simulink model "pole_placement_test"  (R2015b)
settings: Solver=ode3  StartTime=0.0  StopTime=10  FixedStep=0.002  RelTol=1e-3
values from neighbouring files (symbols this model uses):
  k0 = double(poly_coeffs(1))    [pole_placement_script.m]
  k1 = double(poly_coeffs(2))    [pole_placement_script.m]
  k2 = double(poly_coeffs(3))    [pole_placement_script.m]
  k3 = double(poly_coeffs(4))    [pole_placement_script.m]
settings Model: ExtModeTrigDuration=5000  Creator=robertph  LastModifiedBy=robertph
settings SolverCC: PositivePriorityOrder=on
settings RTWCC: SystemTargetFile=quarc_win64.tlc  TemplateMakefile=quarc_default_tmf  Description=QUARC Win64 Target
settings STFCustomTargetCC: GeneratePreprocessorConditionals=Use local settings  CPPClassGenCompliant=off
settings GRTTargetCC: ParMdlRefBuildCompliant=off  CompOptLevelCompliant=off  CombineOutputUpdateFcns=off  MatFileLogging=off  CPPClassGenCompliant=off  GRTInterface=on  UseToolchainInfoCompliant=off  ExtMode=on  ExtModeMexFile=quarc_comm

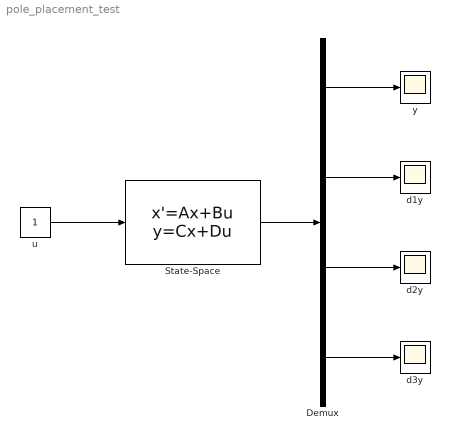
== system pole_placement_test ==
  Demux : Demux
  State-Space : StateSpace  A=[0 1 0 0; 0 0 1 0; 0 0 0 1; -k0, -k1, -k2, -k3]  B=[0; 0; 0; k0]  C=eye(4)  D=zeros(4, 1)  X0=zeros(4, 1)
  d1y : Scope
  d2y : Scope
  d3y : Scope
  u : Constant
  y : Scope
  wires:
  u/1 -> State-Space/1
  State-Space/1 -> Demux/1
  Demux/1 -> y/1
  Demux/2 -> d1y/1
  Demux/3 -> d2y/1
  Demux/4 -> d3y/1
